simulink model "MasseFeder"  (R2024b)
settings: Solver=ode4  StartTime=0.0  StopTime=1000.0  FixedStep=0.001  RelTol=1e-3
settings Model: Creator=root  LastModifiedBy=root

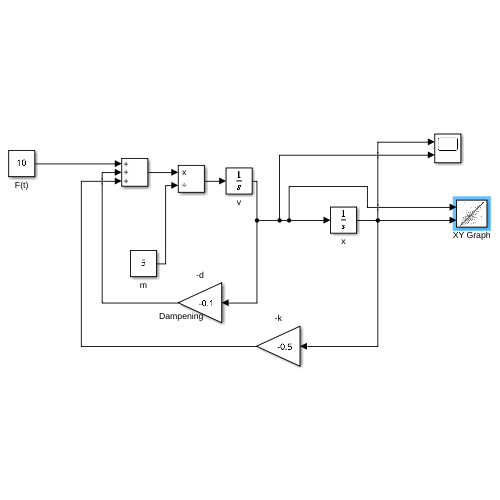
[thumbnail: Simulink's stored preview of the top-level diagram]
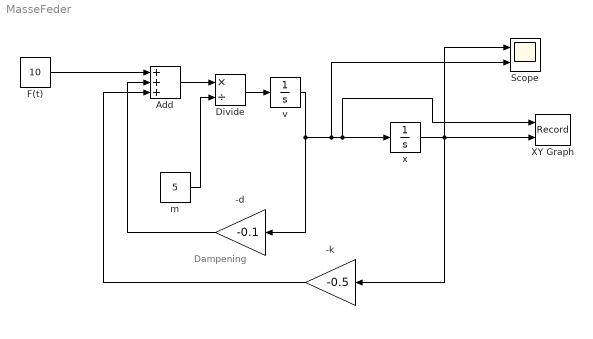
== system MasseFeder ==
  note: Dampening
  -d : Gain  Gain=-0.1
  -k : Gain  Gain=-0.5
  Add : Sum  Inputs=+++
  Divide : Product  Inputs=*/
  F(t) : Constant  Value=10
  Scope : Scope  NumInputPorts=2
  XY Graph : Record  FileSettingsInternal="{\"entries\":[{\"content\":{\"excelSettings\":{\"content\":{},\"type\":\"Streamout.ExcelSettings\"}},\"type\":\"Streamout.FileSettingStorage\",\"uuid\":\"\"}],\"packageUris\":[\"http:\\/\\/schema.mathworks.com\\/mf0\\/streamout_blocks\\/R2020a\"],\"version\":\"1.0\"}"  Layout=[1 1]  SignalsInternal="{\"entries\":[{\"content\":{\"signals\":[{\"content\":{\"blockPath\":[],\"dimensions\":[1],\"domain\":\"\",\"lineColor\":\"#a2142f\",\"plots\":[ 1 ],\"port\":1,\"sid\":[\"\"],\"signalID\":1,\"signalName\":\"v\"},\"type\":\"RecordBlkView.Signal\",\"uuid\":\"\"},{\"content\":{\"blockPath\":[],\"dimensions\":[1],\"domain\":\"\",\"lineColor\":\"#139fff\",\"plots\":[ 1 ],\"port\":2,\"sid\":[\"\"],\"signalID\":2,\"signalName\":\"x\"},\"type\":\"RecordBlkView.Signal\",\"uuid\":\"\"}]},\"type\":\"RecordBlkView.InputSignals\",\"uuid\":\"\"}],\"packageUris\":[\"http:\\/\\/schema.mathworks.com\\/mf0\\/streamout_blocks\\/R2020a\"],\"version\":\"1.0\"}"  VisualizationBindings="{\"xyplotplugin\":{\"info\":[{\"series\":[{\"bindingParametersList\":[{\"parameter\":\"X-Axis\",\"signalID\":1,\"signalName\":\"v\"},{\"parameter\":\"Y-Axis\",\"signalID\":2,\"signalName\":\"x\"}],\"seriesID\":0}],\"subplotID\":1}]}}"  CompatibilityTag=XY
  m : Constant  Value=5
  v : Integrator
  x : Integrator  InitialCondition=10
  wires:
  v/1 -> -d/1, Scope/2, XY Graph/1, x/1
  F(t)/1 -> Add/1
  -k/1 -> Add/3
  Add/1 -> Divide/1
  m/1 -> Divide/2
  Divide/1 -> v/1
  x/1 -> -k/1, XY Graph/2, Scope/1
  -d/1 -> Add/2
